simulink model "Second_Order_System"  (R2012b)
settings: Solver=ode45  StartTime=0.0  StopTime=Tf  MaxStep=1e-5  RelTol=1e-3
values from neighbouring files (symbols this model uses):
  Amp = x(end)    [second_order_driver.m]
  K = 4    [second_order_driver.m]
  omega_n = 0.378    [second_order_driver.m]
  zeta = 0.3965    [second_order_driver.m]
settings Model: Creator=throne  LastModifiedBy=throne
settings DataIOCC: SignalLoggingSaveFormat=ModelDataLogs
settings OptimizationCC: InitFltsAndDblsToZero=on
settings DebuggingCC: FcnCallInpInsideContextMsg=UseLocalSettings  StrictBusMsg=Warning
settings GRTTargetCC: CombineOutputUpdateFcns=off  GRTInterface=on

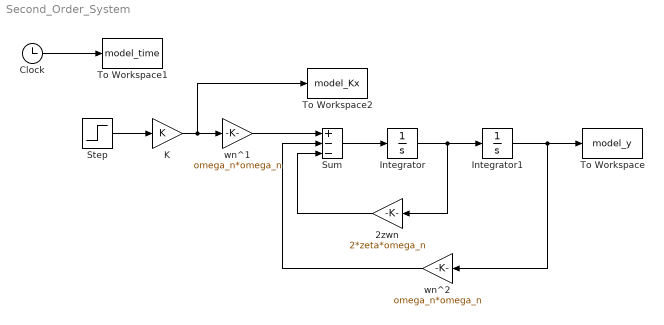
== system Second_Order_System ==
  2zwn : Gain  Gain=2*zeta*omega_n
  Clock : Clock
  Integrator : Integrator
  Integrator1 : Integrator
  K : Gain  Gain=K
  Step : Step  Time=0  After=Amp  SampleTime=0
  Sum : Sum  Inputs=|+|-|-|
  To Workspace : ToWorkspace  VariableName=model_y  SampleTime=-1
  To Workspace1 : ToWorkspace  VariableName=model_time  SampleTime=-1
  To Workspace2 : ToWorkspace  VariableName=model_Kx  SampleTime=-1
  wn^1 : Gain  Gain=omega_n*omega_n
  wn^2 : Gain  Gain=omega_n*omega_n
  wires:
  Sum/1 -> Integrator/1
  Clock/1 -> To Workspace1/1
  Integrator/1 -> Integrator1/1, 2zwn/1
  Integrator1/1 -> To Workspace/1, wn^2/1
  2zwn/1 -> Sum/3
  wn^2/1 -> Sum/2
  Step/1 -> K/1
  wn^1/1 -> Sum/1
  K/1 -> wn^1/1, To Workspace2/1
